simulink model "Lighting_System"  (R2017b)
settings: Solver=VariableStepAuto  StartTime=0.0  StopTime=97  RelTol=1e-3
undefined symbols (not defined in the file): sigbuilder_block
settings Model: Creator=ECoDe_user19  LastModifiedBy=ECoDe_user11
settings DebuggingCC: SignalInfNanChecking=warning  UniqueDataStoreMsg=warning  StrictBusMsg=ErrorOnBusTreatedAsVector
settings ConfigComp: CovEnable=on  RecordCoverage=on  CovMetricSettings=dcmwe  CovModelRefEnable=on

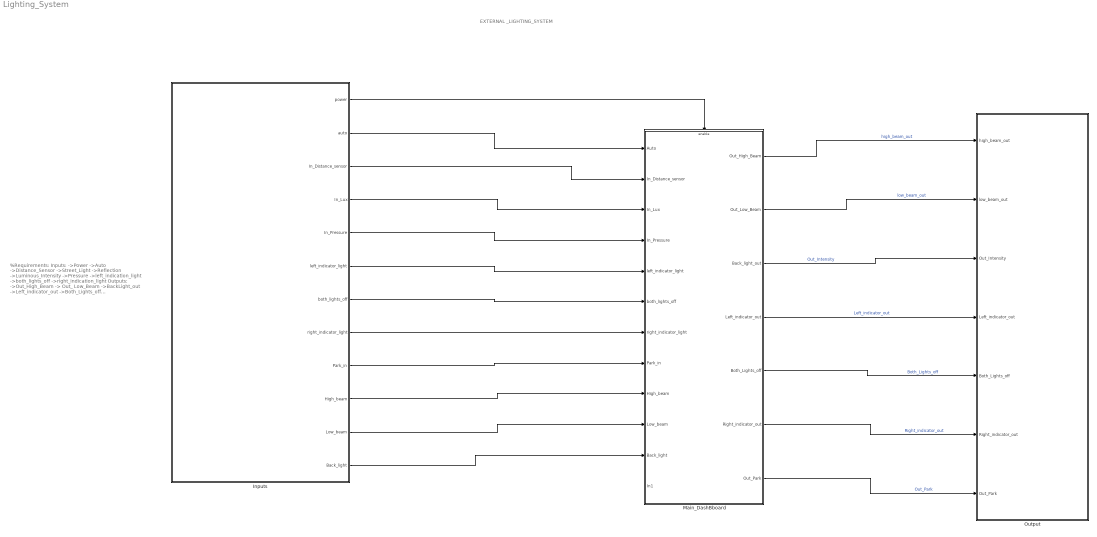
== system Lighting_System ==
  note: EXTERNAL _LIGHTING_SYSTEM
  note: %Requirements:
      | Inputs:
      |
      | ->Power
      | ->Auto
      | ->Distance_Sensor
      | ->Street_Light
      | ->Reflection
      | ->Luminous_Intensity
      | ->Pressure
      | ->left_indication_light
      | ->both_lights_off
      | ->right_indication_light
      | Outputs:
      | ->Out_High_Beam
      | -> Out_ Low_Beam
      | ->BackLight_out
      | ->Left_indicator_out
      | ->Both_Lights_off
      | ->Right_indicator_out
      | ->Indicator Light
  Inputs : Subsystem
  Main_DashBboard : Subsystem
  Output : Subsystem
  wires:
  Main_DashBboard/1(Out_High_Beam) -> Output/1(high_beam_out)  "high_beam_out"
  Main_DashBboard/2(Out_Low_Beam) -> Output/2(low_beam_out)  "low_beam_out"
  Main_DashBboard/3(Back_light_out) -> Output/3(Out_Intensity)  "Out_Intensity"
  Main_DashBboard/4(Left_indicator_out) -> Output/4(Left_indicator_out)  "Left_indicator_out"
  Main_DashBboard/5(Both_Lights_off) -> Output/5(Both_Lights_off)  "Both_Lights_off"
  Main_DashBboard/6(Right_indicator_out) -> Output/6(Right_indicator_out)  "Right_indicator_out"
  Main_DashBboard/7(Out_Park) -> Output/7(Out_Park)  "Out_Park"
  Inputs/1(power) -> Main_DashBboard/Enable
  Inputs/2(auto) -> Main_DashBboard/1(Auto)
  Inputs/3(In_Distance_sensor) -> Main_DashBboard/2(In_Distance_sensor)
  Inputs/4(In_Lux) -> Main_DashBboard/3(In_Lux)
  Inputs/5(In_Pressure) -> Main_DashBboard/4(In_Pressure)
  Inputs/6(left_indicator_light) -> Main_DashBboard/5(left_indicator_light)
  Inputs/7(both_lights_off) -> Main_DashBboard/6(both_lights_off)
  Inputs/8(right_indicator_light) -> Main_DashBboard/7(right_indicator_light)
  Inputs/9(Park_in) -> Main_DashBboard/8(Park_in)
  Inputs/10(High_beam) -> Main_DashBboard/9(High_beam)
  Inputs/11(Low_beam) -> Main_DashBboard/10(Low_beam)
  Inputs/12(Back_light) -> Main_DashBboard/11(Back_light)

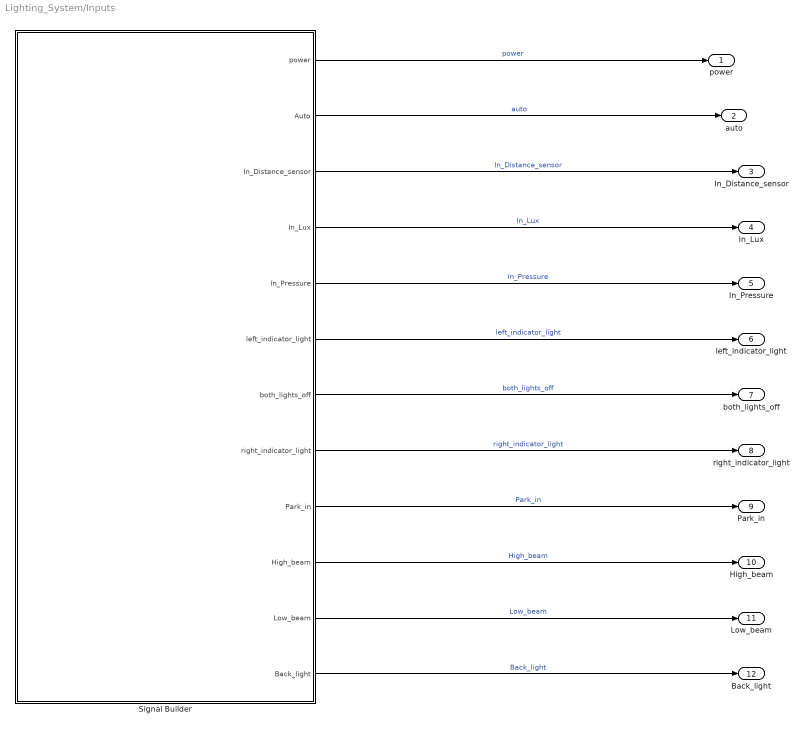
== system Lighting_System/Inputs ==
  Signal Builder : Subsystem  Tag=STV Subsys  LoadFcn=sigbuilder_block('load',[3 36 954 456.75 ]);  StartFcn=sigbuilder_block('start');  StopFcn=sigbuilder_block('stop');  ClipboardFcn=sigbuilder_block('clipboard');  mask(Sigbuilder block){tuvar=[0:10]}
      mask help: Simulink:masks:SigbuilderBlock_MD
      mask init:
      | if ~strcmp(get_param(bdroot(gcbh),'SimulationStatus'),'stopped') tuvar = sigbuilder_block('maskInit'); end
      settings: CopyFcn=sigbuilder_block('copy');  DeleteFcn=sigbuilder_block('delete');  ModelCloseFcn=sigbuilder_block('modelClose');  PreSaveFcn=sigbuilder_block('preSave');  PauseFcn=sigbuilder_block('pause');  ContinueFcn=sigbuilder_block('continue');  NameChangeFcn=sigbuilder_block('namechange');  OpenFcn=sigbuilder_block('open',[3 36 954 456.75 ]);  CloseFcn=sigbuilder_block('close');
      mask Display: plot(0, 0, 100, 100,[2, 2, 32, 32, 2], [68, 8, 8, 68, 68],[32, 2], [38, 38], [32, 19, 2],[53, 60, 44], [32, 17, 17, 2],[16, 16, 31, 31]);txt = getActiveGroup(gcbh);text(2, 100, txt,'verticalAlignment', 'top');
  power : Outport
  auto : Outport  Port=2
  In_Distance_sensor : Outport  Port=3
  In_Lux : Outport  Port=4
  In_Pressure : Outport  Port=5
  left_indicator_light : Outport  Port=6
  both_lights_off : Outport  Port=7
  right_indicator_light : Outport  Port=8
  Park_in : Outport  Port=9
  High_beam : Outport  Port=10
  Low_beam : Outport  Port=11
  Back_light : Outport  Port=12
  wires:
  Signal Builder/4(In_Lux) -> In_Lux/1  "In_Lux"
  Signal Builder/5(In_Pressure) -> In_Pressure/1  "In_Pressure"
  Signal Builder/9(Park_in) -> Park_in/1  "Park_in"
  Signal Builder/8(right_indicator_light) -> right_indicator_light/1  "right_indicator_light"
  Signal Builder/6(left_indicator_light) -> left_indicator_light/1  "left_indicator_light"
  Signal Builder/7(both_lights_off) -> both_lights_off/1  "both_lights_off"
  Signal Builder/3(In_Distance_sensor) -> In_Distance_sensor/1  "In_Distance_sensor"
  Signal Builder/1(power) -> power/1  "power"
  Signal Builder/2(Auto) -> auto/1  "auto"
  Signal Builder/10(High_beam) -> High_beam/1  "High_beam"
  Signal Builder/11(Low_beam) -> Low_beam/1  "Low_beam"
  Signal Builder/12(Back_light) -> Back_light/1  "Back_light"

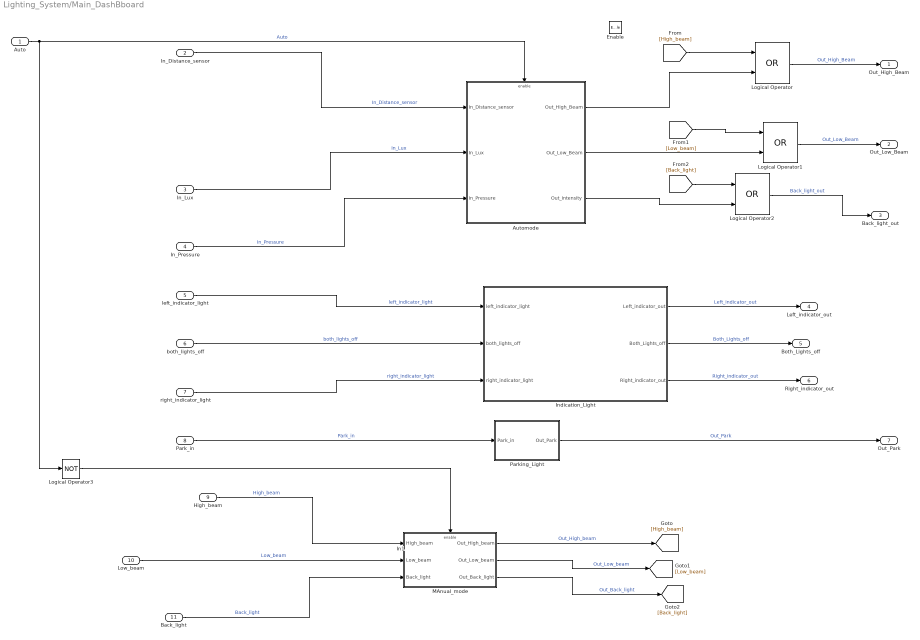
== system Lighting_System/Main_DashBboard ==
  Auto : Inport
  In_Distance_sensor : Inport  Port=2
  In_Lux : Inport  Port=3
  In_Pressure : Inport  Port=4
  left_indicator_light : Inport  Port=5
  both_lights_off : Inport  Port=6
  right_indicator_light : Inport  Port=7
  Park_in : Inport  Port=8
  High_beam : Inport  Port=9
  Low_beam : Inport  Port=10
  Back_light : Inport  Port=11
  In1 : Inport  Port=12
  Enable : EnablePort
  Automode : Subsystem
  Indication_Light : Subsystem
  Logical Operator : Logic  Operator=OR  AllPortsSameDT=off  OutDataTypeStr=boolean
  Logical Operator1 : Logic  Operator=OR  AllPortsSameDT=off  OutDataTypeStr=boolean
  Logical Operator2 : Logic  Operator=OR  AllPortsSameDT=off  OutDataTypeStr=boolean
  Logical Operator3 : Logic  Operator=NOT  AllPortsSameDT=off  OutDataTypeStr=boolean
  MAnual_mode : Subsystem
  Parking_Light : Subsystem
  Out_High_Beam : Outport
  Out_Low_Beam : Outport  Port=2
  Back_light_out : Outport  Port=3
  Left_indicator_out : Outport  Port=4
  Both_Lights_off : Outport  Port=5
  Right_indicator_out : Outport  Port=6
  Out_Park : Outport  Port=7
  wires:
  both_lights_off/1 -> Indication_Light/2(both_lights_off)  "both_lights_off"
  left_indicator_light/1 -> Indication_Light/1(left_indicator_light)  "left_indicator_light"
  Park_in/1 -> Parking_Light/1(Park_in)  "Park_in"
  Parking_Light/1(Out_Park) -> Out_Park/1  "Out_Park"
  right_indicator_light/1 -> Indication_Light/3(right_indicator_light)  "right_indicator_light"
  Indication_Light/1(Left_indicator_out) -> Left_indicator_out/1  "Left_indicator_out"
  Indication_Light/2(Both_Lights_off) -> Both_Lights_off/1  "Both_Lights_off"
  Indication_Light/3(Right_indicator_out) -> Right_indicator_out/1  "Right_indicator_out"
  In_Distance_sensor/1 -> Automode/1(In_Distance_sensor)  "In_Distance_sensor"
  In_Lux/1 -> Automode/2(In_Lux)  "In_Lux"
  In_Pressure/1 -> Automode/3(In_Pressure)  "In_Pressure"
  Auto/1 -> Automode/Enable, Logical Operator3/1  "Auto"
  [High_beam] -> Logical Operator/1
  Automode/1(Out_High_Beam) -> Logical Operator/2
  Logical Operator/1 -> Out_High_Beam/1  "Out_High_Beam"
  Automode/2(Out_Low_Beam) -> Logical Operator1/2
  [Low_beam] -> Logical Operator1/1
  Logical Operator1/1 -> Out_Low_Beam/1  "Out_Low_Beam"
  [Back_light] -> Logical Operator2/1
  Automode/3(Out_Intensity) -> Logical Operator2/2
  Logical Operator2/1 -> Back_light_out/1  "Back_light_out"
  High_beam/1 -> MAnual_mode/1(High_beam)  "High_beam"
  Low_beam/1 -> MAnual_mode/2(Low_beam)  "Low_beam"
  Back_light/1 -> MAnual_mode/3(Back_light)  "Back_light"
  MAnual_mode/1(Out_High_beam) -> [High_beam]  "Out_High_beam"
  MAnual_mode/2(Out_Low_beam) -> [Low_beam]  "Out_Low_beam"
  MAnual_mode/3(Out_Back_light) -> [Back_light]  "Out_Back_light"
  Logical Operator3/1 -> MAnual_mode/Enable

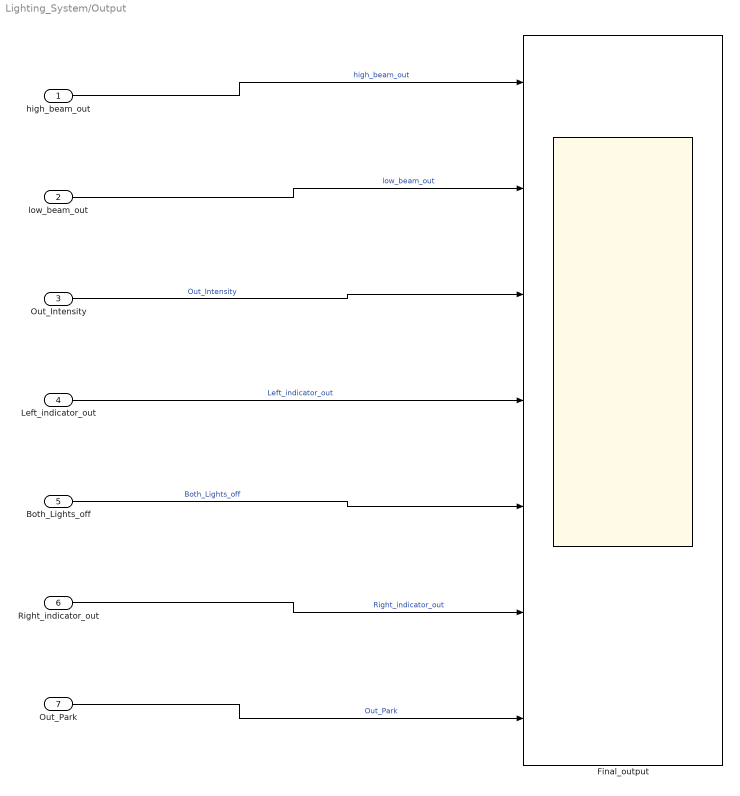
== system Lighting_System/Output ==
  high_beam_out : Inport
  low_beam_out : Inport  Port=2
  Out_Intensity : Inport  Port=3
  Left_indicator_out : Inport  Port=4
  Both_Lights_off : Inport  Port=5
  Right_indicator_out : Inport  Port=6
  Out_Park : Inport  Port=7
  Final_output : Scope  NumInputPorts=7
  wires:
  high_beam_out/1 -> Final_output/1  "high_beam_out"
  Out_Park/1 -> Final_output/7  "Out_Park"
  low_beam_out/1 -> Final_output/2  "low_beam_out"
  Out_Intensity/1 -> Final_output/3  "Out_Intensity"
  Left_indicator_out/1 -> Final_output/4  "Left_indicator_out"
  Right_indicator_out/1 -> Final_output/6  "Right_indicator_out"
  Both_Lights_off/1 -> Final_output/5  "Both_Lights_off"

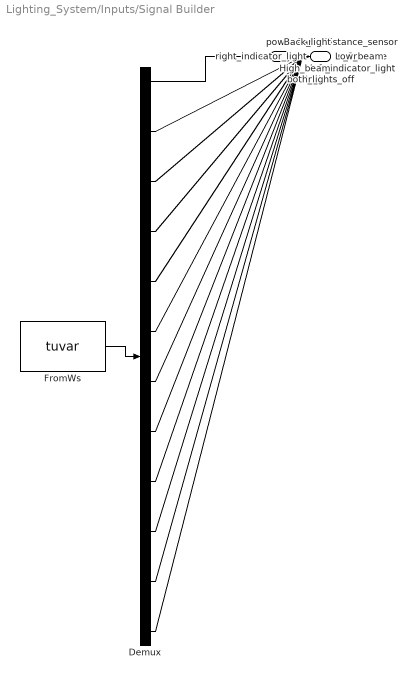
== system Lighting_System/Inputs/Signal Builder ==
  Demux : Demux  Tag=STV Demux  Outputs=12
  FromWs : FromWorkspace  Tag=STV FromWs  VariableName=tuvar  SampleTime=0
      SigBuilderData=|
      | common.afterFinalStr = 'Extrapolate'
      | common.sampleTime = 0
      | dataSet.timeRange = [0 97]
      | dataSet.name = 'Sheet1'
      | sbobj.Name = 'Signal Builder'
      | sbobj.Groups.Name = 'Sheet1'
      | sbobj.Groups.Signals(1).Name = 'power'
      | sbobj.Groups.Signals(1).XData = [0 1 2 3 4 5 6 7 8 9 10 11 12 13 14 15 16 17 18 19 20 21 22 23 24 25 26 27 28 29 30 31 32 33 34 35 36 37 38 39 40 41 42 43 44 45 46 47 48 49 50 51 52 53 54 55 56 57 58 59 60 61 62 63 64 65 66 67 68 69 70 71 72 73 74 75 76 77 78 79 80 81 82 83 84 85 86 87 88 89 90 91 92 93 94 95 96 97]
      | sbobj.Groups.Signals(1).YData = [1 1 1 1 1 1 1 1 1 1 1 1 1 1 1 1 1 1 1 1 1 1 1 1 1 1 1 1 1 1 1 1 1 1 1 1 1 1 1 1 1 1 1 1 1 1 1 1 1 1 1 1 1 1 1 1 1 1 1 1 1 1 1 1 1 1 1 1 1 1 1 1 1 1 1 1 1 1 1 1 1 1 1 1 1 1 1 1 1 1 1 1 1 1 1 1 1 1]
      | sbobj.Groups.Signals(2).Name = 'Auto'
      | sbobj.Groups.Signals(2).XData = [0 1 2 3 4 5 6 7 8 9 10 11 12 13 14 15 16 17 18 19 20 21 22 23 24 25 26 27 28 29 30 31 32 33 34 35 36 37 38 39 40 41 42 43 44 45 46 47 48 49 50 51 52 53 54 55 56 57 58 59 60 61 62 63 64 65 66 67 68 69 70 71 72 73 74 75 76 77 78 79 80 81 82 83 84 85 86 87 88 89 90 91 92 93 94 95 96 97]
      | sbobj.Groups.Signals(2).YData = [1 1 1 1 1 1 1 1 1 1 1 1 1 1 1 1 1 1 1 1 1 1 1 1 1 1 1 1 1 1 1 1 1 1 1 1 1 1 1 1 1 1 1 1 1 1 1 1 1 1 1 1 1 1 1 1 1 1 1 1 1 1 1 1 1 1 1 1 1 1 1 1 1 1 1 1 1 1 1 1 1 1 1 1 1 1 1 1 0 0 0 0 0 0 0 0 0 0]
      | sbobj.Groups.Signals(3).Name = 'In_Distance_sensor'
      | sbobj.Groups.Signals(3).XData = [0 1 2 3 4 5 6 7 8 9 10 11 12 13 14 15 16 17 18 19 20 21 22 23 24 25 26 27 28 29 30 31 32 33 34 35 36 37 38 39 40 41 42 43 44 45 46 47 48 49 50 51 52 53 54 55 56 57 58 59 60 61 62 63 64 65 66 67 68 69 70 71 72 73 74 75 76 77 78 79 80 81 82 83 84 85 86 87 88 89 90 91 92 93 94 95 96 97]
      | sbobj.Groups.Signals(3).YData = [0 15 4 4 16 28 4 6 28 20 4 27 16 47 46.5 46 30 28 26 24 22 20 18 16 14 12 10 8 6 5 4.5 4 3.5 3 2.5 2 1.5 1 0.5 0 53 53 54 55 56 56 0 0 0 15 4 4 16 28 4 6 28 20 4 27 16 53 54 55 56 66 24 24 24 24 23 22 21 20 19 18 17 16 15 14 13 12 0 0 0 0 0 56 0 0 0 0 0 0 0 0 0 0]
      | sbobj.Groups.Signals(4).Name = 'In_Lux'
      | sbobj.Groups.Signals(4).XData = [0 1 2 3 4 5 6 7 8 9 10 11 12 13 14 15 16 17 18 19 20 21 22 23 24 25 26 27 28 29 30 31 32 33 34 35 36 37 38 39 40 41 42 43 44 45 46 47 48 49 50 51 52 53 54 55 56 57 58 59 60 61 62 63 64 65 66 67 68 69 70 71 72 73 74 75 76 77 78 79 80 81 82 83 84 85 86 87 88 89 90 91 92 93 94 95 96 97]
      | sbobj.Groups.Signals(4).YData = [1 1 5 10 15 20 25 30 35 40 45 50 55 60 65 70 75 80 85 90 95 100 105 110 115 120 125 130 135 140 145 150 155 160 165 170 175 180 185 190 30 30 90 360 450 450 0 0 0 1 5 10 15 1 5 10 15 1 5 10 15 1 5 10 15 1 5 5 5 5 35 40 45 50 35 40 45 50 35 40 45 50 50 35 40 45 50 80 0 0 0 0 0 0 0 0 0 0]
      | sbobj.Groups.Signals(5).Name = 'In_Pressure'
      | sbobj.Groups.Signals(5).XData = [0 1 2 3 4 5 6 7 8 9 10 11 12 13 14 15 16 17 18 19 20 21 22 23 24 25 26 27 28 29 30 31 32 33 34 35 36 37 38 39 40 41 42 43 44 45 46 47 48 49 50 51 52 53 54 55 56 57 58 59 60 61 62 63 64 65 66 67 68 69 70 71 72 73 74 75 76 77 78 79 80 81 82 83 84 85 86 87 88 89 90 91 92 93 94 95 96 97]
      | sbobj.Groups.Signals(5).YData = [35 35 10 180 65 12 15 18 21 24 27 30 33 36 39 40 50 60 70 80 90 100 110 120 130 140 150 160 170 180 190 200 210 220 230 240 250 260 270 280 30 35 60 90 120 120 0 0 0 0 3 6 9 12 15 18 0 3 6 9 12 35 10 180 65 30 200 250 150 180 12 15 18 21 24 15 18 21 24 15 18 21 21 24 15 18 21 65 0 0 0 0 0 0 0 0 0 0]
      | sbobj.Groups.Signals(6).Name = 'left_indicator_light'
      | sbobj.Groups.Signals(6).XData = [0 1 2 3 4 5 6 7 8 9 10 11 12 13 14 15 16 17 18 19 20 21 22 23 24 25 26 27 28 29 30 31 32 33 34 35 36 37 38 39 40 41 42 43 44 45 46 47 48 49 50 51 52 53 54 55 56 57 58 59 60 61 62 63 64 65 66 67 68 69 70 71 72 73 74 75 76 77 78 79 80 81 82 83 84 85 86 87 88 89 90 91 92 93 94 95 96 97]
      | sbobj.Groups.Signals(6).YData = [1 1 1 1 1 0 0 0 0 0 0 0 0 0 0 1 1 1 1 1 0 0 0 0 0 0 0 0 0 0 1 1 1 1 1 0 0 0 0 0 0 0 0 0 0 1 1 1 1 1 0 0 0 0 0 0 0 0 0 0 1 1 1 1 1 0 0 0 0 0 0 0 0 0 0 1 1 1 1 1 0 0 0 0 0 0 0 0 0 0 0 0 0 1 1 1 1 1]
      | sbobj.Groups.Signals(7).Name = 'both_lights_off'
      | sbobj.Groups.Signals(7).XData = [0 1 2 3 4 5 6 7 8 9 10 11 12 13 14 15 16 17 18 19 20 21 22 23 24 25 26 27 28 29 30 31 32 33 34 35 36 37 38 39 40 41 42 43 44 45 46 47 48 49 50 51 52 53 54 55 56 57 58 59 60 61 62 63 64 65 66 67 68 69 70 71 72 73 74 75 76 77 78 79 80 81 82 83 84 85 86 87 88 89 90 91 92 93 94 95 96 97]
      | sbobj.Groups.Signals(7).YData = [0 0 0 0 0 0 0 0 0 0 1 1 1 1 1 0 0 0 0 0 0 0 0 0 0 1 1 1 1 1 0 0 0 0 0 0 0 0 0 0 1 1 1 1 1 0 0 0 0 0 0 0 0 0 0 1 1 1 1 1 0 0 0 0 0 0 0 0 0 0 1 1 1 1 1 0 0 0 0 0 0 0 0 0 0 1 1 1 1 1 1 1 1 0 0 0 0 0]
      | sbobj.Groups.Signals(8).Name = 'right_indicator_light'
      | sbobj.Groups.Signals(8).XData = [0 1 2 3 4 5 6 7 8 9 10 11 12 13 14 15 16 17 18 19 20 21 22 23 24 25 26 27 28 29 30 31 32 33 34 35 36 37 38 39 40 41 42 43 44 45 46 47 48 49 50 51 52 53 54 55 56 57 58 59 60 61 62 63 64 65 66 67 68 69 70 71 72 73 74 75 76 77 78 79 80 81 82 83 84 85 86 87 88 89 90 91 92 93 94 95 96 97]
      | sbobj.Groups.Signals(8).YData = [0 0 0 0 0 1 1 1 1 1 0 0 0 0 0 0 0 0 0 0 1 1 1 1 1 0 0 0 0 0 0 0 0 0 0 1 1 1 1 1 0 0 0 0 0 0 0 0 0 0 1 1 1 1 1 0 0 0 0 0 0 0 0 0 0 1 1 1 1 1 0 0 0 0 0 0 0 0 0 0 1 1 1 1 1 0 0 0 0 0 0 0 0 0 0 0 0 0]
      | sbobj.Groups.Signals(9).Name = 'Park_in'
      | sbobj.Groups.Signals(9).XData = [0 1 2 3 4 5 6 7 8 9 10 11 12 13 14 15 16 17 18 19 20 21 22 23 24 25 26 27 28 29 30 31 32 33 34 35 36 37 38 39 40 41 42 43 44 45 46 47 48 49 50 51 52 53 54 55 56 57 58 59 60 61 62 63 64 65 66 67 68 69 70 71 72 73 74 75 76 77 78 79 80 81 82 83 84 85 86 87 88 89 90 91 92 93 94 95 96 97]
      | sbobj.Groups.Signals(9).YData = [0 0 0 0 0 0 0 0 0 0 0 0 0 0 0 0 0 0 0 0 0 0 0 0 0 0 0 0 0 0 0 0 0 0 0 0 0 0 0 0 0 0 0 0 1 1 1 1 1 0 0 0 0 0 0 0 0 0 0 0 0 0 0 0 0 0 0 0 0 0 0 0 0 0 0 0 0 0 0 0 0 0 0 0 0 0 0 0 0 0 0 0 0 0 0 0 0 0]
      | sbobj.Groups.Signals(10).Name = 'High_beam'
      | sbobj.Groups.Signals(10).XData = [0 1 2 3 4 5 6 7 8 9 10 11 12 13 14 15 16 17 18 19 20 21 22 23 24 25 26 27 28 29 30 31 32 33 34 35 36 37 38 39 40 41 42 43 44 45 46 47 48 49 50 51 52 53 54 55 56 57 58 59 60 61 62 63 64 65 66 67 68 69 70 71 72 73 74 75 76 77 78 79 80 81 82 83 84 85 86 87 88 89 90 91 92 93 94 95 96 97]
      | sbobj.Groups.Signals(10).YData = [0 0 0 0 0 0 0 0 0 0 0 0 0 0 0 0 0 0 0 0 0 0 0 0 0 0 0 0 0 0 0 0 0 0 0 0 0 0 0 0 0 0 0 0 0 0 0 0 0 0 0 0 0 0 0 0 0 0 0 0 0 0 0 0 0 0 0 0 0 0 0 0 0 0 0 0 0 0 0 0 0 0 0 0 0 0 0 0 1 1 1 1 1 1 0 0 0 0]
      | sbobj.Groups.Signals(11).Name = 'Low_beam'
      | sbobj.Groups.Signals(11).XData = [0 1 2 3 4 5 6 7 8 9 10 11 12 13 14 15 16 17 18 19 20 21 22 23 24 25 26 27 28 29 30 31 32 33 34 35 36 37 38 39 40 41 42 43 44 45 46 47 48 49 50 51 52 53 54 55 56 57 58 59 60 61 62 63 64 65 66 67 68 69 70 71 72 73 74 75 76 77 78 79 80 81 82 83 84 85 86 87 88 89 90 91 92 93 94 95 96 97]
      | sbobj.Groups.Signals(11).YData = [0 0 0 0 0 0 0 0 0 0 0 0 0 0 0 0 0 0 0 0 0 0 0 0 0 0 0 0 0 0 0 0 0 0 0 0 0 0 0 0 0 0 0 0 0 0 0 0 0 0 0 0 0 0 0 0 0 0 0 0 0 0 0 0 0 0 0 0 0 0 0 0 0 0 0 0 0 0 0 0 0 0 0 0 0 0 0 0 1 1 1 1 0 0 1 1 1 1]
      | sbobj.Groups.Signals(12).Name = 'Back_light'
      | sbobj.Groups.Signals(12).XData = [0 1 2 3 4 5 6 7 8 9 10 11 12 13 14 15 16 17 18 19 20 21 22 23 24 25 26 27 28 29 30 31 32 33 34 35 36 37 38 39 40 41 42 43 44 45 46 47 48 49 50 51 52 53 54 55 56 57 58 59 60 61 62 63 64 65 66 67 68 69 70 71 72 73 74 75 76 77 78 79 80 81 82 83 84 85 86 87 88 89 90 91 92 93 94 95 96 97]
      | sbobj.Groups.Signals(12).YData = [0 0 0 0 0 0 0 0 0 0 0 0 0 0 0 0 0 0 0 0 0 0 0 0 0 0 0 0 0 0 0 0 0 0 0 0 0 0 0 0 0 0 0 0 0 0 0 0 0 0 0 0 0 0 0 0 0 0 0 0 0 0 0 0 0 0 0 0 0 0 0 0 0 0 0 0 0 0 0 0 0 0 0 0 0 0 0 0 1 1 1 1 0 0 1 1 0 0]
      | sbobj.Groups.TimeRange = [0 97]
  power : Outport  Tag=STV Outport
  Auto : Outport  Tag=STV Outport  Port=2
  In_Distance_sensor : Outport  Tag=STV Outport  Port=3
  In_Lux : Outport  Tag=STV Outport  Port=4
  In_Pressure : Outport  Tag=STV Outport  Port=5
  left_indicator_light : Outport  Tag=STV Outport  Port=6
  both_lights_off : Outport  Tag=STV Outport  Port=7
  right_indicator_light : Outport  Tag=STV Outport  Port=8
  Park_in : Outport  Tag=STV Outport  Port=9
  High_beam : Outport  Tag=STV Outport  Port=10
  Low_beam : Outport  Tag=STV Outport  Port=11
  Back_light : Outport  Tag=STV Outport  Port=12
  wires:
  Demux/1 -> power/1
  FromWs/1 -> Demux/1
  Demux/2 -> Auto/1
  Demux/3 -> In_Distance_sensor/1
  Demux/4 -> In_Lux/1
  Demux/5 -> In_Pressure/1
  Demux/6 -> left_indicator_light/1
  Demux/7 -> both_lights_off/1
  Demux/8 -> right_indicator_light/1
  Demux/9 -> Park_in/1
  Demux/10 -> High_beam/1
  Demux/11 -> Low_beam/1
  Demux/12 -> Back_light/1

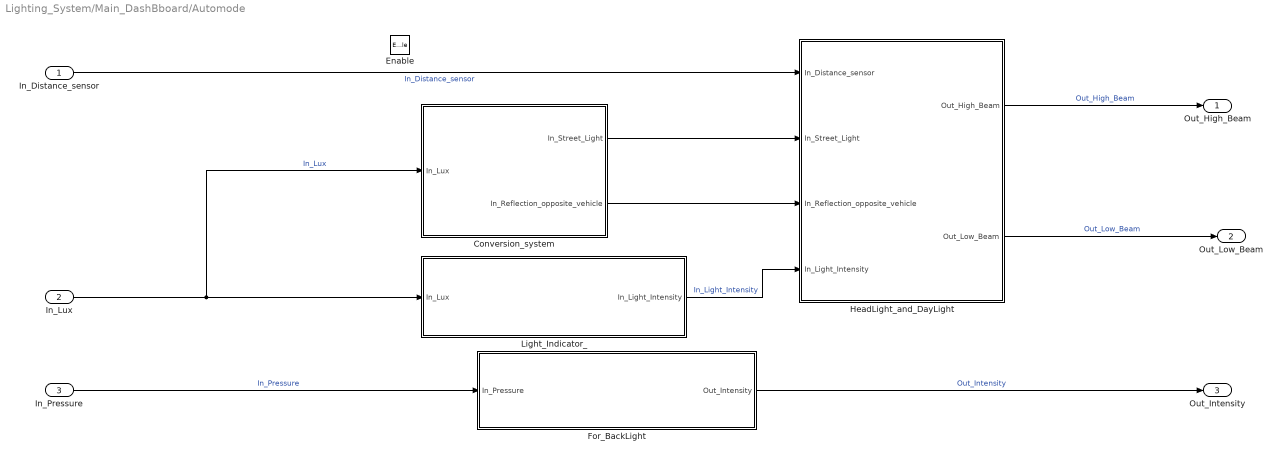
== system Lighting_System/Main_DashBboard/Automode ==
  In_Distance_sensor : Inport
  In_Lux : Inport  Port=2
  In_Pressure : Inport  Port=3
  Enable : EnablePort
  Conversion_system : Subsystem
  For_BackLight : Subsystem
  HeadLight_and_DayLight : Subsystem
  Light_Indicator_ : Subsystem
  Out_High_Beam : Outport
  Out_Low_Beam : Outport  Port=2
  Out_Intensity : Outport  Port=3
  wires:
  For_BackLight/1(Out_Intensity) -> Out_Intensity/1  "Out_Intensity"
  In_Lux/1 -> Conversion_system/1(In_Lux), Light_Indicator_/1(In_Lux)  "In_Lux"
  HeadLight_and_DayLight/2(Out_Low_Beam) -> Out_Low_Beam/1  "Out_Low_Beam"
  In_Pressure/1 -> For_BackLight/1(In_Pressure)  "In_Pressure"
  In_Distance_sensor/1 -> HeadLight_and_DayLight/1(In_Distance_sensor)  "In_Distance_sensor"
  HeadLight_and_DayLight/1(Out_High_Beam) -> Out_High_Beam/1  "Out_High_Beam"
  Light_Indicator_/1(In_Light_Intensity) -> HeadLight_and_DayLight/4(In_Light_Intensity)  "In_Light_Intensity"
  Conversion_system/2(In_Reflection_opposite_vehicle) -> HeadLight_and_DayLight/3(In_Reflection_opposite_vehicle)
  Conversion_system/1(In_Street_Light) -> HeadLight_and_DayLight/2(In_Street_Light)

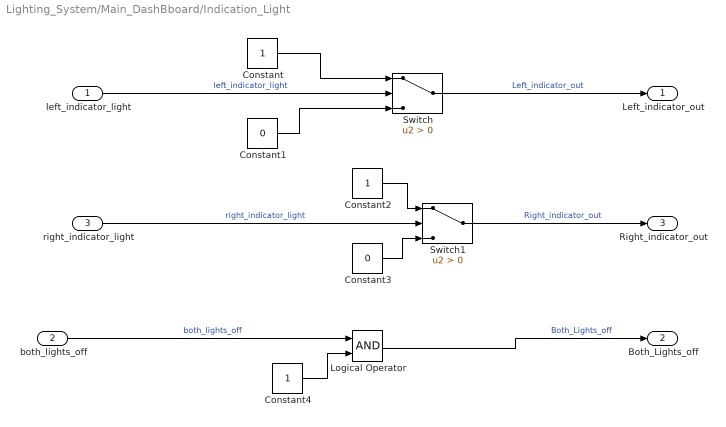
== system Lighting_System/Main_DashBboard/Indication_Light ==
  left_indicator_light : Inport
  both_lights_off : Inport  Port=2
  right_indicator_light : Inport  Port=3
  Constant : Constant
  Constant1 : Constant  Value=0
  Constant2 : Constant
  Constant3 : Constant  Value=0
  Constant4 : Constant
  Logical Operator : Logic  AllPortsSameDT=off  OutDataTypeStr=boolean
  Switch : Switch  Criteria=u2 > Threshold
  Switch1 : Switch  Criteria=u2 > Threshold
  Left_indicator_out : Outport
  Both_Lights_off : Outport  Port=2
  Right_indicator_out : Outport  Port=3
  wires:
  left_indicator_light/1 -> Switch/2  "left_indicator_light"
  Constant/1 -> Switch/1
  Constant1/1 -> Switch/3
  Constant3/1 -> Switch1/3
  right_indicator_light/1 -> Switch1/2  "right_indicator_light"
  Constant2/1 -> Switch1/1
  Switch/1 -> Left_indicator_out/1  "Left_indicator_out"
  Switch1/1 -> Right_indicator_out/1  "Right_indicator_out"
  Constant4/1 -> Logical Operator/2
  both_lights_off/1 -> Logical Operator/1  "both_lights_off"
  Logical Operator/1 -> Both_Lights_off/1  "Both_Lights_off"

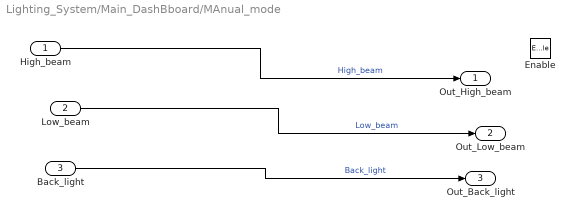
== system Lighting_System/Main_DashBboard/MAnual_mode ==
  High_beam : Inport
  Low_beam : Inport  Port=2
  Back_light : Inport  Port=3
  Enable : EnablePort
  Out_High_beam : Outport
  Out_Low_beam : Outport  Port=2
  Out_Back_light : Outport  Port=3
  wires:
  High_beam/1 -> Out_High_beam/1  "High_beam"
  Low_beam/1 -> Out_Low_beam/1  "Low_beam"
  Back_light/1 -> Out_Back_light/1  "Back_light"

== system Lighting_System/Main_DashBboard/Parking_Light ==
  Park_in : Inport
  Compare_with_Light : Switch  Criteria=u2 > Threshold
  Lower_Limit : Constant  Value=0
  Out_Park : Outport
  wires:
  Park_in/1 -> Compare_with_Light/1, Compare_with_Light/2  "Park_in"
  Lower_Limit/1 -> Compare_with_Light/3  "Lower_Limit"
  Compare_with_Light/1 -> Out_Park/1  "Out_Park"

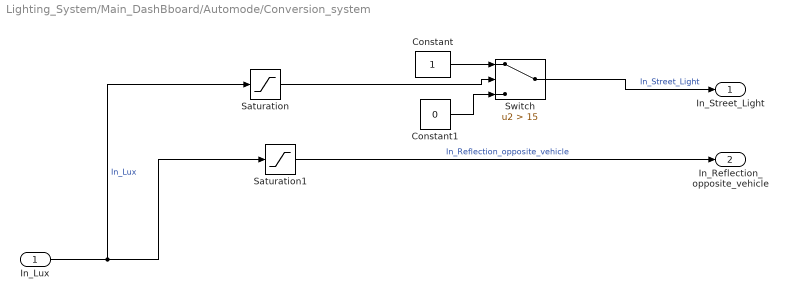
== system Lighting_System/Main_DashBboard/Automode/Conversion_system ==
  In_Lux : Inport
  Constant : Constant
  Constant1 : Constant  Value=0
  Saturation : Saturate  UpperLimit=20  LowerLimit=10
      settings: AttributesFormatString=|
      | %<UpperLimit>
      | %<LowerLimit>
  Saturation1 : Saturate  UpperLimit=200  LowerLimit=150
      settings: AttributesFormatString=|
      | %<UpperLimit>
      | %<LowerLimit>
  Switch : Switch  Criteria=u2 > Threshold  Threshold=15
      settings: AttributesFormatString=%<Threshold>
  In_Street_Light : Outport
  In_Reflection_opposite_vehicle : Outport  Port=2
  wires:
  Constant1/1 -> Switch/3
  Switch/1 -> In_Street_Light/1  "In_Street_Light"
  Saturation/1 -> Switch/2
  Constant/1 -> Switch/1
  Saturation1/1 -> In_Reflection_opposite_vehicle/1  "In_Reflection_opposite_vehicle"
  In_Lux/1 -> Saturation1/1, Saturation/1  "In_Lux"

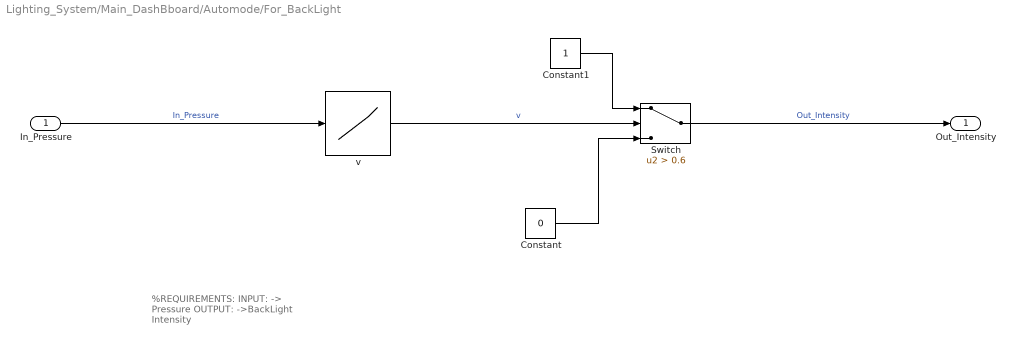
== system Lighting_System/Main_DashBboard/Automode/For_BackLight ==
  note: %REQUIREMENTS:
      | INPUT:
      | -> Pressure
      | OUTPUT:
      | ->BackLight Intensity
  In_Pressure : Inport
  Constant : Constant  Value=0
  Constant1 : Constant
  Switch : Switch  Criteria=u2 > Threshold  Threshold=0.6
      settings: AttributesFormatString=%<Threshold>
  v : Lookup_n-D  NumberOfTableDimensions=1  BreakpointsForDimension1=[0 300]  Table=[0 5]  InternalRulePriority=Speed  RndMeth=Simplest  InputSameDT=on
      settings: AttributesFormatString=%<RndMeth>Floor
  Out_Intensity : Outport
  wires:
  v/1 -> Switch/2  "v"
  In_Pressure/1 -> v/1  "In_Pressure"
  Switch/1 -> Out_Intensity/1  "Out_Intensity"
  Constant1/1 -> Switch/1
  Constant/1 -> Switch/3

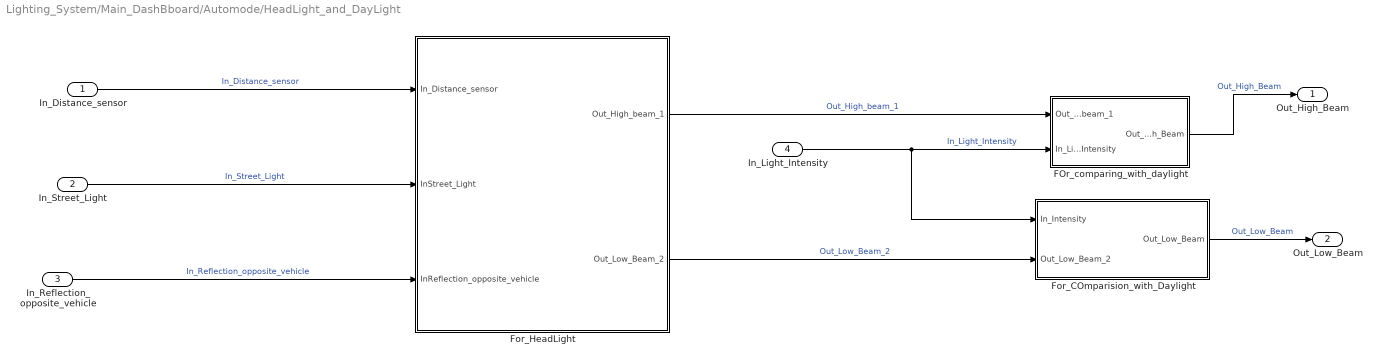
== system Lighting_System/Main_DashBboard/Automode/HeadLight_and_DayLight ==
  In_Distance_sensor : Inport
  In_Street_Light : Inport  Port=2
  In_Reflection_opposite_vehicle : Inport  Port=3
  In_Light_Intensity : Inport  Port=4
  FOr_comparing_with_daylight : Subsystem
  For_COmparision_with_Daylight : Subsystem
  For_HeadLight : Subsystem
  Out_High_Beam : Outport
  Out_Low_Beam : Outport  Port=2
  wires:
  In_Light_Intensity/1 -> For_COmparision_with_Daylight/1(In_Intensity), FOr_comparing_with_daylight/2(In_Light_Intensity)  "In_Light_Intensity"
  In_Street_Light/1 -> For_HeadLight/2(InStreet_Light)  "In_Street_Light"
  In_Reflection_opposite_vehicle/1 -> For_HeadLight/3(InReflection_opposite_vehicle)  "In_Reflection_opposite_vehicle"
  In_Distance_sensor/1 -> For_HeadLight/1(In_Distance_sensor)  "In_Distance_sensor"
  For_HeadLight/1(Out_High_beam_1) -> FOr_comparing_with_daylight/1(Out_High_beam_1)  "Out_High_beam_1"
  FOr_comparing_with_daylight/1(Out_High_Beam) -> Out_High_Beam/1  "Out_High_Beam"
  For_HeadLight/2(Out_Low_Beam_2) -> For_COmparision_with_Daylight/2(Out_Low_Beam_2)  "Out_Low_Beam_2"
  For_COmparision_with_Daylight/1(Out_Low_Beam) -> Out_Low_Beam/1  "Out_Low_Beam"

== system Lighting_System/Main_DashBboard/Automode/Light_Indicator_ ==
  note: %REQUIREMENTS:
      | Input:
      | ->Luminous_intensity
      | Output:
      | ->Maintainable_Intensity
  In_Lux : Inport
  Day_light_intense : Stateflow chart  TreatAsAtomicUnit=on
  f : Lookup_n-D  NumberOfTableDimensions=1  BreakpointsForDimension1=[0 800]  Table=[0 3]  InternalRulePriority=Speed  RndMeth=Simplest  InputSameDT=on
      settings: AttributesFormatString=%<RndMeth>Floor
  In_Light_Intensity : Outport
  wires:
  Day_light_intense/1(In_Light_Intensity) -> In_Light_Intensity/1  "In_Light_Intensity"
  In_Lux/1 -> f/1  "In_Lux"
  f/1 -> Day_light_intense/1(f)  "f"

== system Lighting_System/Main_DashBboard/Automode/HeadLight_and_DayLight/FOr_comparing_with_daylight ==
  Out_High_beam_1 : Inport
  In_Light_Intensity : Inport  Port=2
  Compare_with_Daylight2 : RelationalOperator  OutDataTypeStr=boolean  RndMeth=Simplest
  Out_High_Beam : Outport
  wires:
  Out_High_beam_1/1 -> Compare_with_Daylight2/1  "Out_High_beam_1"
  Compare_with_Daylight2/1 -> Out_High_Beam/1  "Out_High_Beam"
  In_Light_Intensity/1 -> Compare_with_Daylight2/2  "In_Light_Intensity"

== system Lighting_System/Main_DashBboard/Automode/HeadLight_and_DayLight/For_COmparision_with_Daylight ==
  In_Intensity : Inport
  Out_Low_Beam_2 : Inport  Port=2
  Compare_with_Daylight : RelationalOperator  OutDataTypeStr=boolean  RndMeth=Simplest
  Out_Low_Beam : Outport
  wires:
  In_Intensity/1 -> Compare_with_Daylight/2  "In_Intensity"
  Out_Low_Beam_2/1 -> Compare_with_Daylight/1  "Out_Low_Beam_2"
  Compare_with_Daylight/1 -> Out_Low_Beam/1  "Out_Low_Beam"

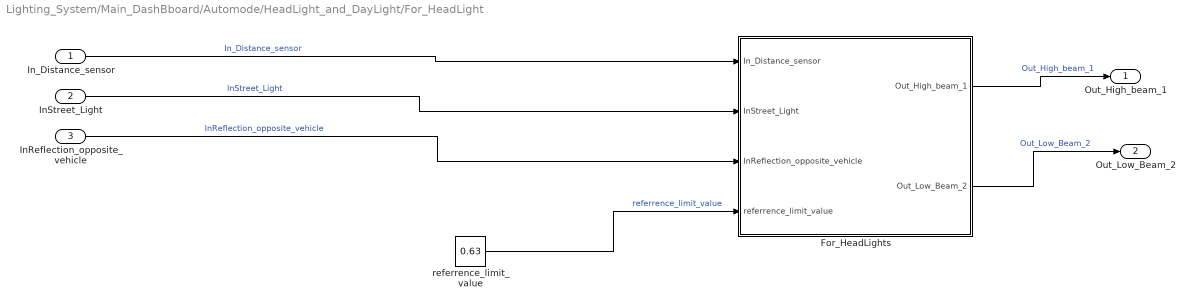
== system Lighting_System/Main_DashBboard/Automode/HeadLight_and_DayLight/For_HeadLight ==
  In_Distance_sensor : Inport
  InStreet_Light : Inport  Port=2
  InReflection_opposite_vehicle : Inport  Port=3
  For_HeadLights : Stateflow chart  TreatAsAtomicUnit=on
  referrence_limit_value : Constant  Value=0.63
  Out_High_beam_1 : Outport
  Out_Low_Beam_2 : Outport  Port=2
  wires:
  InStreet_Light/1 -> For_HeadLights/2(InStreet_Light)  "InStreet_Light"
  In_Distance_sensor/1 -> For_HeadLights/1(In_Distance_sensor)  "In_Distance_sensor"
  InReflection_opposite_vehicle/1 -> For_HeadLights/3(InReflection_opposite_vehicle)  "InReflection_opposite_vehicle"
  referrence_limit_value/1 -> For_HeadLights/4(referrence_limit_value)  "referrence_limit_value"
  For_HeadLights/2(Out_Low_Beam_2) -> Out_Low_Beam_2/1  "Out_Low_Beam_2"
  For_HeadLights/1(Out_High_beam_1) -> Out_High_beam_1/1  "Out_High_beam_1"

== stateflow chart Lighting_System/Main_DashBboard/Automode/HeadLight_and_DayLight/For_HeadLight/For_HeadLights ==
  state High_beam
    en:
    st=1;
    du:
    Out_High_beam_1=1;
    Out_Low_Beam_2=1;
  state Low_decrease
    en:
    st=2;
    du:
    Out_High_beam_1=0;
    Out_Low_Beam_2=In_Distance_sensor/25;
  state Low_turn_off
    en:
    st=4;
    du:
    Out_High_beam_1=0;
    Out_Low_Beam_2=0;
  state Low_beam
    en:
    st=3;
    du:
    Out_High_beam_1=0;
    Out_Low_Beam_2=1;
  note: % Requirements:
      | Inputs:
      | -> ux:Obstacle Distance sensing
      | ->uy: Reflection of the car opposite
      | ->uz: Street_Light_Detection
      | ->u_limit:Reflection light limit
      | Outputs:
      | ->u1:High Beam
      | ->u2:Low Beam
      | Logic:
      | ->When the obstacle is greater than 25 meters and Street_Light_Detection is less than 1 then the high beam,Low beam is turned ON
      | ->When the obstacle 5 to 25 meters the high beam is turned OFF and low beam is turned ON.Intensity depending on distance
      | ->When Obstacle is less than 5 meters and Street_Light_Detection is greater than 1 then Low beam Turned 'ON'
      | -> If Reflection light limit is more than the considered limit then turn off
      | low beam and if less turn on low beam
  High_beam -> Low_beam [order 2] : [In_Distance_sensor<=5 & InStreet_Light<1]
  High_beam -> Low_beam [order 3] : [InStreet_Light>=1]
  (default) -> High_beam
  Low_beam -> High_beam [order 2] : [In_Distance_sensor>50 & InStreet_Light<1]
  Low_decrease -> High_beam [order 2] : [In_Distance_sensor>25  & InStreet_Light<1]
  High_beam -> Low_decrease [order 1] : [In_Distance_sensor>5 &In_Distance_sensor<=25]
  Low_turn_off -> High_beam [order 3] : [In_Distance_sensor>25 & InStreet_Light<1]
  Low_beam -> Low_turn_off [order 3] : [InReflection_opposite_vehicle>referrence_limit_value &In_Distance_sensor<=5]
  Low_decrease -> Low_beam [order 3] : [In_Distance_sensor>5 & InStreet_Light>=1]
  Low_turn_off -> Low_beam [order 1] : [InReflection_opposite_vehicle<referrence_limit_value & In_Distance_sensor <=5]
  Low_beam -> Low_decrease [order 1] : [In_Distance_sensor>5&In_Distance_sensor<=25]
  Low_decrease -> Low_beam [order 1] : [In_Distance_sensor<=5]
  Low_turn_off -> Low_decrease [order 2] : [In_Distance_sensor>5 & In_Distance_sensor <=25]
  data: In_Distance_sensor input; Out_High_beam_1 output; Out_Low_Beam_2 output; InStreet_Light input; InReflection_opposite_vehicle input; referrence_limit_value input; st local

== stateflow chart Lighting_System/Main_DashBboard/Automode/Light_Indicator_/Day_light_intense ==
  state Sun_rise_set
    en:
    In_Light_Intensity=0.25;
  state night
    en:
    In_Light_Intensity=0.5;
  state Sunny
    en:
    In_Light_Intensity=0;
  state Dark_night
    en:
    In_Light_Intensity=1;
  note: %REQUIREMENTS:
      | Input:
      | ->f-Luminous intensity
      | Output:
      | ->Int-Intensity Maintainable
  (default) -> Sun_rise_set
  night -> Sun_rise_set : [f<1.5 && f>1]
  Sun_rise_set -> Sunny : [f>1.5]
  Sunny -> night [order 1] : [f>0.2 && f <1]
  Sunny -> Dark_night [order 2] : [f<0.2]
  Dark_night -> Sunny : [f>0.2]
  data: f input; In_Light_Intensity output
